simulink model "RIN251129_16_18_14_L3"  (R2018b)
settings: Solver=FixedStepAuto  StartTime=0.0  StopTime=0.05  RelTol=1e-3
libraries: powerlib x49, powerlib_meascontrol x17
settings Model: Creator=ADMINISTRATOR  LastModifiedBy=VID Company
settings SFSimCC: SimUseLocalCustomCode=off
settings RTWCC: RTWUseLocalCustomCode=off
settings CodeAppCC: StateflowObjectComments=on
settings SimscapeCC: SimscapeNormalizeSystem=off

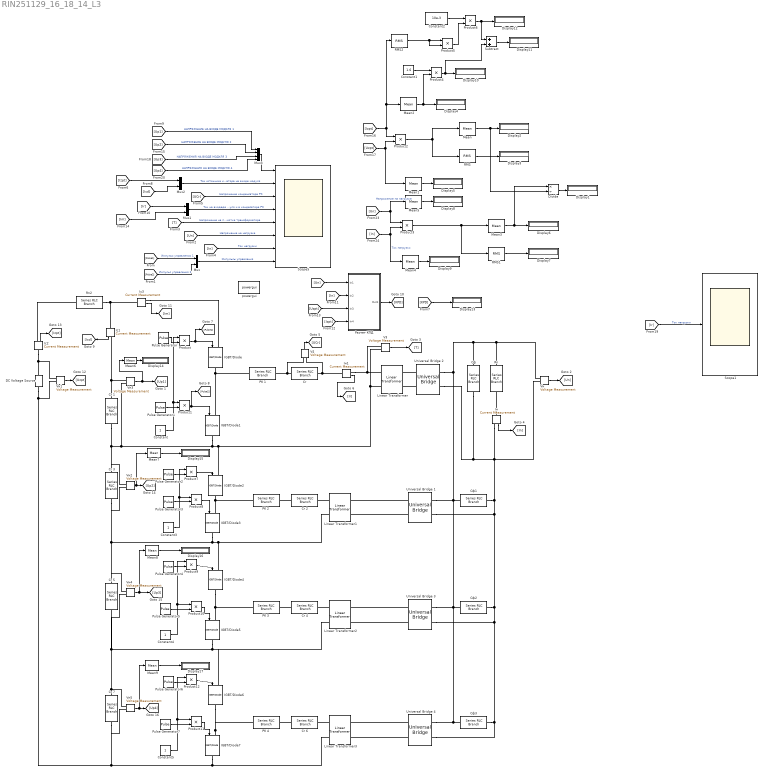
== system RIN251129_16_18_14_L3 ==
  " Rn" : powerlib/Elements/Series RLC Branch  LConnTagsString=__new0  RConnTagsString=__new0  BranchType=R  Resistance=2.3  Inductance=1e-3  SetiL0=off  InitialCurrent=0  Capacitance=1e-6  Setx0=off  InitialVoltage=0  Measurements=Branch voltage and current
      settings: SourceProductName=Simscape Electrical
  " Rn2" : powerlib/Elements/Series RLC Branch  LConnTagsString=__new0  RConnTagsString=__new0  BranchType=RL  Resistance=6  Inductance=1e-6  SetiL0=off  InitialCurrent=0  Capacitance=1e-6  Setx0=off  InitialVoltage=0  Measurements=Branch voltage and current
      settings: SourceProductName=Simscape Electrical
  Constant{,3..5} (4 alike) : Constant
  Constant1 : Constant  Value=1.6
  Constant2 : Constant  Value=10e-3
  Cr {,2,4,6} (4 alike) : powerlib/Elements/Series RLC Branch  LConnTagsString=__new0  RConnTagsString=__new0  BranchType=C  Resistance=0.001  Inductance=5e-6  SetiL0=off  InitialCurrent=0  Capacitance=1.6e-6  Setx0=off  InitialVoltage=0  Measurements=Branch voltage and current
      settings: SourceProductName=Simscape Electrical
  Cr {1,3,5,7} (4 alike) : powerlib/Elements/Series RLC Branch  LConnTagsString=__new0  RConnTagsString=__new0  BranchType=C  Resistance=0.00005  Inductance=5e-6  SetiL0=off  InitialCurrent=0  Capacitance=20e-6  Setx0=off  InitialVoltage=0  Measurements=Branch voltage and current
      settings: SourceProductName=Simscape Electrical
  DC Voltage Source : powerlib/Electrical Sources/DC Voltage Source  Amplitude=2020  Measurements=None
      settings: SourceProductName=Simscape Electrical
  Display{1..17} (17 alike) : Display
  Divide : Product  Inputs=*/
  IGBT/Diode{,1..7} (8 alike) : powerlib/Power Electronics/IGBT//Diode  Ron=4.5e-6  Rs=1e5  Cs=inf  Measurements=off
      settings: SourceProductName=Simscape Electrical
  Ic1 : powerlib/Measurements/Current Measurement  PhasorSimulation=off  OutputType=Complex  PSBequivalent=0
      settings: SourceProductName=Simscape Electrical
  Ic2 : powerlib/Measurements/Current Measurement  PhasorSimulation=off  OutputType=Complex  PSBequivalent=0
      settings: SourceProductName=Simscape Electrical
  Ic3 : powerlib/Measurements/Current Measurement  PhasorSimulation=off  OutputType=Complex  PSBequivalent=0
      settings: SourceProductName=Simscape Electrical
  Iн : powerlib/Measurements/Current Measurement  PhasorSimulation=off  OutputType=Complex  PSBequivalent=0
      settings: SourceProductName=Simscape Electrical
  Iн1 : powerlib/Measurements/Current Measurement  PhasorSimulation=off  OutputType=Complex  PSBequivalent=0
      settings: SourceProductName=Simscape Electrical
  Linear Transformer{,1..3} (4 alike) : powerlib/Elements/Linear Transformer  UNITS=pu  NominalPower=[ 2e3 7e4 ]  winding1=[250 1e-4 1e-7]  winding2=[325 1e-4 1e-7]  ThreeWindings=off  winding3=[3.15e+05 0.7938 0.084225]  RmLm=[1e4 1e4]  Measurements=None  DataType=off
      settings: SourceProductName=Simscape Electrical
  Mean{,1..9} (10 alike) : powerlib_meascontrol/Measurements/Mean  Freq=16e3  Vinit=0  Ts=0
      settings: SourceProductName=Simscape Electrical
  Mux : Mux  Inputs=2
  Mux1 : Mux  Inputs=2
  Mux2 : Mux  Inputs=2
  Mux3 : Mux
  Product{,1..12} (13 alike) : Product
  Pulse Generator : DiscretePulseGenerator  PulseType=Time based  Amplitude=20  Period=1/16e3  PulseWidth=27
  Pulse Generator1 : DiscretePulseGenerator  PulseType=Time based  Amplitude=20  Period=1/16e3  PulseWidth=27  PhaseDelay=1/32e3
  Pulse Generator2 : DiscretePulseGenerator  PulseType=Time based  Amplitude=20  Period=1/16e3  PulseWidth=27  PhaseDelay=1/16e3/4
  Pulse Generator3 : DiscretePulseGenerator  PulseType=Time based  Amplitude=20  Period=1/16e3  PulseWidth=27  PhaseDelay=1/32e3 + 1/16e3/4
  Pulse Generator4 : DiscretePulseGenerator  PulseType=Time based  Amplitude=20  Period=1/16e3  PulseWidth=27  PhaseDelay=1/16e3/2
  Pulse Generator5 : DiscretePulseGenerator  PulseType=Time based  Amplitude=20  Period=1/16e3  PulseWidth=27  PhaseDelay=1/32e3 + 1/16e3/2
  Pulse Generator6 : DiscretePulseGenerator  PulseType=Time based  Amplitude=20  Period=1/16e3  PulseWidth=27  PhaseDelay=3/16e3/8
  Pulse Generator7 : DiscretePulseGenerator  PulseType=Time based  Amplitude=20  Period=1/16e3  PulseWidth=27  PhaseDelay=1/32e3 + 3/16e3/8
  RMS : powerlib_meascontrol/Measurements/RMS  TrueRMS=on  Freq=16e3  RMSInit=0  Ts=0
      settings: SourceProductName=Simscape Electrical
  RMS1 : powerlib_meascontrol/Measurements/RMS  TrueRMS=on  Freq=16e3  RMSInit=0  Ts=0
      settings: SourceProductName=Simscape Electrical
  RMS2 : powerlib_meascontrol/Measurements/RMS  TrueRMS=on  Freq=16e3  RMSInit=0  Ts=0
      settings: SourceProductName=Simscape Electrical
  Scope1 : Scope
  Scope5 : Scope  NumInputPorts=8
  Subtract : Sum
  Universal Bridge {1..4} (4 alike) : powerlib/Power Electronics/Universal Bridge  Arms=2  SnubberResistance=1000000  SnubberCapacitance=1e-12  Device=Diodes  Ron=1e-6  Lon=0  ForwardVoltages="[  0  0  ]"  ForwardVoltage=0  GTOparameters=[ 10e-6 , 20e-6 ]  IGBTparameters=[ 1e-6 , 2e-6 ]  Measurements=None  Measurements_2=None  converterType=Rectifier
      settings: SourceProductName=Simscape Electrical
  V3 : powerlib/Measurements/Voltage Measurement  PhasorSimulation=off  OutputType=Complex  PSBequivalent=0
      settings: SourceProductName=Simscape Electrical
  V4 : powerlib/Measurements/Voltage Measurement  PhasorSimulation=off  OutputType=Complex  PSBequivalent=0
      settings: SourceProductName=Simscape Electrical
  Vн{,1..5} (6 alike) : powerlib/Measurements/Voltage Measurement  PhasorSimulation=off  OutputType=Complex  PSBequivalent=0
      settings: SourceProductName=Simscape Electrical
  powergui : powerlib/powergui  Priority=1  SimulationMode=Discrete  SampleTime=1e-7  frequency=60  Iterations=50  frequencyindice=0  Pbase=100e6  ErrMax=1e-4  UnitsV=kV  UnitsW=MW  buscounter=0  FunctionMessages=off  echomessages=off  EnableUseOfTLC=off  CurrentSourceSwitches=off  DisableSnubberDevices=off  DisableRonSwitches=off  DisableVfSwitches=off  DisplayEquations=off  SolverType=Tustin/Backward Euler (TBE)  Interpol=off  ExternalGateDelay=off  methode=off  Ts=100  x0status=blocks  SPID=off  SwTol=0  HookPort=off  RestoreLinks=warning  ResistiveCurrentMeasurement=off  Frange=[0:2:500]  Ylog=off  Xlog=on  ShowGrid=off  save=off  variable=ZData  structure=0  ZoomFFT=off  StartTime=0.0  cycles=1  DisplayStyle=1  fundamental=60  FreqAxis=off  MaxFrequency=1000  frequencyindicesteady=1  RmsSteady=1  display=off
  РК {1..4} (4 alike) : powerlib/Elements/Series RLC Branch  LConnTagsString=__new0  RConnTagsString=__new0  BranchType=RL  Resistance=0.000001  Inductance=13.6e-6  SetiL0=off  InitialCurrent=0  Capacitance=3e-6  Setx0=off  InitialVoltage=0  Measurements=None
      settings: SourceProductName=Simscape Electrical
  Расчет КПД : Subsystem
  Сф{,1..3} (4 alike) : powerlib/Elements/Series RLC Branch  LConnTagsString=__new0  RConnTagsString=__new0  BranchType=C  Resistance=0.001  Inductance=5e-6  SetiL0=off  InitialCurrent=0  Capacitance=120e-6  Setx0=off  InitialVoltage=300  Measurements=Branch voltage and current
      settings: SourceProductName=Simscape Electrical
  wires:
  Vн/1 -> [Un]
  V3/1 -> [T]
  Iн/1 -> [In]
  V4/1 -> [UCr]
  [UCr] -> Scope5/3  "Напряжение конденсатора РК"
  Iн1/1 -> [Ir]
  [In] -> Scope5/7  "Ток нагрузки"
  [Un] -> Scope5/6  "Напряжение на нагрузке"
  [T] -> Scope5/5  "Напряжение на первичной обмотке трансформатора"
  Product1/1 -> IGBT/Diode1/1, [Pulse2]
  Product/1 -> [Pulse1], IGBT/Diode/1
  [Un] -> Расчет КПД/1(In1)
  [In] -> Расчет КПД/2(In2)
  [Uzpt] -> Расчет КПД/3(In3)
  [Izpt] -> Расчет КПД/4(In4)
  Расчет КПД/1(Out1) -> [KPD]
  Pulse Generator/1 -> Product/2
  Pulse Generator1/1 -> Product1/2
  Constant/1 -> Product/1, Product1/1
  [Izpt] -> Product2/1, Mean2/1, RMS2/1
  [Uzpt] -> Product2/2, Mean1/1
  Product2/1 -> RMS/1, Mean/1
  RMS/1 -> Display3/1
  Mean1/1 -> Display5/1
  Mean2/1 -> Product4/2, Display4/1
  Product3/1 -> RMS1/1, Mean3/1
  RMS1/1 -> Display7/1
  Mean3/1 -> Divide/1, Display6/1
  Mean4/1 -> Display9/1
  Mean5/1 -> Display8/1
  [Un] -> Mean5/1, Product3/1  "Напряжение на нагрузке"
  [In] -> Product3/2, Mean4/1  "Ток нагрузки"
  Divide/1 -> Display1/1
  Mean/1 -> Divide/2, Display2/1
  Constant1/1 -> Product4/1
  RMS2/1 -> Product5/1, Product5/2
  Constant2/1 -> Product6/1
  Product5/1 -> Product6/2
  Product6/1 -> Display12/1, Subtract/1
  Product4/1 -> Subtract/2, Display10/1
  Subtract/1 -> Display11/1
  Mux2/1 -> Scope5/2  "Ток источника и конденсатора на входе модуля"
  Vн3/1 -> Mean6/1, [Up1]
  [Pulse1] -> Mux/1  "Импульс управления 1"
  [Pulse2] -> Mux/2  "Импульс управления 2"
  Product8/1 -> IGBT/Diode3/1
  Product7/1 -> IGBT/Diode2/1
  Pulse Generator2/1 -> Product7/2
  Pulse Generator3/1 -> Product8/2
  Constant3/1 -> Product7/1, Product8/1
  Ic1/1 -> [Icd]
  Ic2/1 -> [Izpt]
  Ic3/1 -> [Im]
  [Ir] -> Mux1/1
  [Im] -> Mux1/2
  Mux1/1 -> Scope5/4  "Ток на входеде модуля и в кондесаторе РК"
  [Izpt] -> Mux2/1
  Mux/1 -> Scope5/8  "Импульсы управления"
  Vн1/1 -> [Uzpt]
  [KPD] -> Display13/1
  Vн2/1 -> Mean7/1, [Up2]
  [Up2] -> Mux3/2  "НАПРЯЖЕНИЕ НА ВХОДЕ МОДУЛЯ 2"
  [Up1] -> Mux3/1  "НАПРЯЖЕНИЕ НА ВХОДЕ МОДУЛЯ 1"
  Mux3/1 -> Scope5/1
  Product10/1 -> IGBT/Diode5/1
  Pulse Generator4/1 -> Product9/2
  Pulse Generator5/1 -> Product10/2
  Constant4/1 -> Product9/1, Product10/1
  Vн4/1 -> Mean8/1, [Up3]
  [Up3] -> Mux3/3  "НАПРЯЖЕНИЯ НА ВХОДЕ МОДУЛЯ 3"
  Product9/1 -> IGBT/Diode4/1
  Mean8/1 -> Display16/1
  Mean7/1 -> Display15/1
  Mean6/1 -> Display14/1
  [Ir] -> Scope1/1  "Ток нагрузки"
  Pulse Generator6/1 -> Product12/2
  Product12/1 -> IGBT/Diode6/1
  Constant5/1 -> Product12/1, Product11/1
  Pulse Generator7/1 -> Product11/2
  Vн5/1 -> Mean9/1, [Up4]
  Mean9/1 -> Display17/1
  Product11/1 -> IGBT/Diode7/1
  [Icd] -> Mux2/2
  [Up4] -> Mux3/4  "НАПРЯЖЕНИЯ НА ВХОДЕ МОДУЛЯ 4"
  connections:
  РК 1/LConn1 -- IGBT/Diode1/LConn1 -- IGBT/Diode/RConn1
  "Cr "/RConn1 -- V4/LConn2 -- Iн1/LConn1
  Universal Bridge 4/RConn1 -- Vн/LConn1 -- " Rn"/LConn1 -- Сф/LConn1 -- Universal Bridge 2/RConn1 -- Сф1/RConn1 -- Universal Bridge 1/RConn1 -- Сф2/RConn1 -- Universal Bridge 3/RConn1 -- Сф3/RConn1
  Iн/LConn1 -- " Rn"/RConn1
  V4/LConn1 -- "Cr "/LConn1 -- РК 1/RConn1
  Iн1/RConn1 -- Linear Transformer/LConn1 -- V3/LConn1
  Universal Bridge 4/RConn2 -- Сф/RConn1 -- Universal Bridge 2/RConn2 -- Vн/LConn2 -- Iн/RConn1 -- Сф1/LConn1 -- Universal Bridge 1/RConn2 -- Сф2/LConn1 -- Universal Bridge 3/RConn2 -- Сф3/LConn1
  Cr 1/RConn1 -- Cr 3/LConn1 -- Vн2/LConn1 -- Vн3/LConn2 -- IGBT/Diode2/LConn1 -- Linear Transformer/LConn2 -- V3/LConn2 -- IGBT/Diode1/RConn1
  Universal Bridge 2/LConn2 -- Linear Transformer/RConn2
  Universal Bridge 2/LConn1 -- Linear Transformer/RConn1
  " Rn2"/LConn1 -- Ic3/LConn1 -- Ic1/LConn1
  IGBT/Diode2/RConn1 -- IGBT/Diode3/LConn1 -- РК 2/LConn1
  Cr 2/LConn1 -- РК 2/RConn1
  Universal Bridge 1/LConn2 -- Linear Transformer1/RConn2
  Universal Bridge 1/LConn1 -- Linear Transformer1/RConn1
  Linear Transformer1/LConn1 -- Cr 2/RConn1
  Cr 1/LConn1 -- Vн3/LConn1 -- Ic1/RConn1
  Ic2/LConn1 -- Vн1/LConn1 -- DC Voltage Source/RConn1
  Ic2/RConn1 -- " Rn2"/RConn1
  Ic3/RConn1 -- IGBT/Diode/LConn1
  РК 3/LConn1 -- IGBT/Diode4/RConn1 -- IGBT/Diode5/LConn1
  Vн5/LConn1 -- Cr 7/LConn1 -- Cr 5/RConn1 -- Vн4/LConn2 -- IGBT/Diode6/LConn1 -- Linear Transformer2/LConn2 -- IGBT/Diode5/RConn1
  Universal Bridge 3/LConn1 -- Linear Transformer2/RConn1
  Universal Bridge 3/LConn2 -- Linear Transformer2/RConn2
  Cr 4/LConn1 -- РК 3/RConn1
  Linear Transformer2/LConn1 -- Cr 4/RConn1
  Linear Transformer1/LConn2 -- Cr 5/LConn1 -- Vн4/LConn1 -- Cr 3/RConn1 -- Vн2/LConn2 -- IGBT/Diode3/RConn1 -- IGBT/Diode4/LConn1
  IGBT/Diode7/LConn1 -- РК 4/LConn1 -- IGBT/Diode6/RConn1
  DC Voltage Source/LConn1 -- IGBT/Diode7/RConn1 -- Linear Transformer3/LConn2 -- Cr 7/RConn1 -- Vн5/LConn2 -- Vн1/LConn2
  Linear Transformer3/LConn1 -- Cr 6/RConn1
  Universal Bridge 4/LConn2 -- Linear Transformer3/RConn2
  Universal Bridge 4/LConn1 -- Linear Transformer3/RConn1
  Cr 6/LConn1 -- РК 4/RConn1

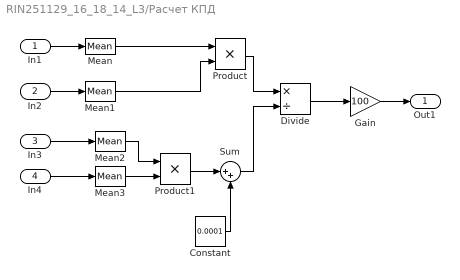
== system RIN251129_16_18_14_L3/Расчет КПД ==
  In1 : Inport
  In2 : Inport  Port=2
  In3 : Inport  Port=3
  In4 : Inport  Port=4
  Constant : Constant  Value=0.0001
  Divide : Product  Inputs=*/
  Gain : Gain  Gain=100
  Mean{,1..3} (4 alike) : powerlib_meascontrol/Measurements/Mean  Freq=16e3  Vinit=0  Ts=0
      settings: SourceProductName=Simscape Electrical
  Product : Product
  Product1 : Product
  Sum : Sum  Inputs=|++
  Out1 : Outport
  wires:
  Product/1 -> Divide/1
  Divide/1 -> Gain/1
  Gain/1 -> Out1/1
  In1/1 -> Mean/1
  Mean/1 -> Product/1
  In2/1 -> Mean1/1
  Mean1/1 -> Product/2
  In3/1 -> Mean2/1
  Mean2/1 -> Product1/1
  In4/1 -> Mean3/1
  Mean3/1 -> Product1/2
  Product1/1 -> Sum/1
  Sum/1 -> Divide/2
  Constant/1 -> Sum/2
